simulink model "frequency_measurement_withHELP"  (R2013a)
settings: Solver=ode45  StartTime=0.0  StopTime=0.1  RelTol=1e-3
PreLoadFcn:
  | Freq=[0 150;1 150];
InitFcn:
  | Freq=[0 150;1 150];
  | hit=0.00001;
  | v=.1;
libraries: simulink x1, dspswit3 x1, dspsigops x1
settings Model: Creator=MAT-DEPT  LastModifiedBy=CYBORG
settings DataIOCC: SignalLoggingSaveFormat=ModelDataLogs
settings OptimizationCC: ExpressionDepthLimit=2147483647
settings DebuggingCC: FcnCallInpInsideContextMsg=UseLocalSettings  StrictBusMsg=Warning
settings GRTTargetCC: CombineOutputUpdateFcns=off  GRTInterface=on

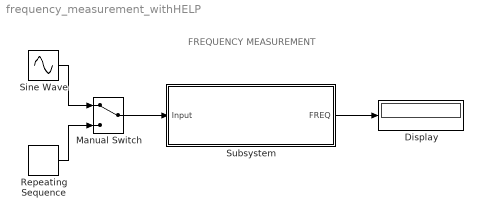
== system frequency_measurement_withHELP ==
  note: FREQUENCY MEASUREMENT
  Display : Display
  Manual Switch : ManualSwitch
  Repeating Sequence : simulink/Sources/Repeating Sequence  rep_seq_t=[0 1/3000]  rep_seq_y=[0 1]
  Sine Wave : Sin  Frequency=2*pi*30  SampleTime=0
  Subsystem : Subsystem  mask(Frequency Measurement){b=External Signal, a=Freq, fo=500, hit=.5, v=0.1}
      mask prompts: b "Type of input:"; a "Workspace Data Identifier:"; fo "Test Frequency fo(Hz)"; hit "Hit value for the Non Zero-Crossing signals:"; v "Time scaling factor:"
      mask help:
      | This block measures the frequency of the input signal, also the workspace signal.
      | User can even check the block using the TEST SIGNAL checkbox.
      mask Help:
      | This block measures the frequency of the input signal, also the workspace signal.
      | User can even check the block using the TEST SIGNAL checkbox.
      | </br>
      | <b></br><h3><u>PARAMETERS</u></h3></b></br>
      | <b><u>Type of input:</u></b></br>
      | <b>1.External Signal:</b>To check the frequency of a external signal, Connect the signal to the 'Input' port of the block.</br>
      | <b></br><u>Workspace Data Identifier</u></b></br>There comes a situation where the model runs too slow. In such sitations or a predefined Workspace data set '2' in <b>Type of input</b> and give the workspace variable name.</br> Model initializes with a workspace variable of 'Freq'. User can specify their own Identifier in <b>Workspace Data Identifier</b></br></br>
      | <b><u>Use TEST SIGNAL</u></b></br>Inorder to test the block check the <b>Use TEST SIGNAL</b> check box.
      | </br><b><u></br>Test Frequency f0(Hz):</u></b></br>Specify the frequency of the test signal in <b>Test Frequency f0(Hz)</b>
      | </br></br><b><u>Hit value for the Non Zero-Crossing signals:</u></b></br>
      | The model uses a zero crossing hit detector with rising edge to count the signal .So if the given input signal is not crossing and rising from zero the counter cannot count the exact cycles. So it is recommended to give the center amplitude value of the given signal to get the proper output.
      | </br></br><i><h2><font color='orange'>Note:</font><font color='brown'> The Frequncy will be found after 1 second, because </br><align='center'><b>Frequency = Number of cycles per second.</b></align></font> </marque></font></h2></i></br>
      mask TypeOptions b: External Signal | Workspace Data | Test Signal
      mask Callback b: b_cb(gcb)
      mask Display:
      | disp('FREQUENCY')
      | port_label('input', 1, 'Input')
      | port_label('output', 1, 'Freq')
  wires:
  Subsystem/1(FREQ) -> Display/1
  Sine Wave/1 -> Manual Switch/1
  Repeating Sequence/1 -> Manual Switch/2
  Manual Switch/1 -> Subsystem/1(Input)

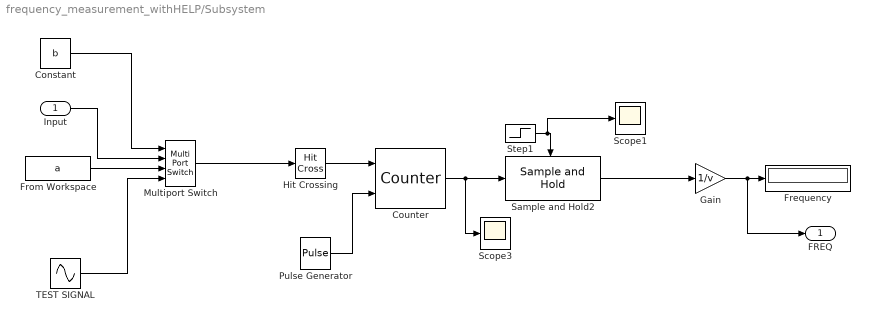
== system frequency_measurement_withHELP/Subsystem ==
  Input : Inport
  Constant : Constant  Value=b
  Counter : dspswit3/Counter  Direction=Up  CountEvent=Rising edge  CounterSize=User defined  MaxCount=10000  InitialCount=0  Output=Count  HitValue=32  ResetInput=on  SamplesPerFrame=1  Ts=1  CntDtype=double  HitDtype=Logical
  "Frequency " : Display
  From Workspace : FromWorkspace  VariableName=a  SampleTime=0
  Gain : Gain  Gain=1/v
  Hit Crossing : HitCross  HitCrossingOffset=hit  HitCrossingDirection=rising
  Multiport Switch : MultiPortSwitch
  Pulse Generator : DiscretePulseGenerator  PulseType=Time based  Period=1  PhaseDelay=v
  Sample and Hold2 : dspsigops/Sample and Hold  trig=Rising edge  initCond=0  latchinput=off
  Scope1 : Scope
      settings: YMin=0  YMax=70  SampleInput=on  SampleTime=5e-6
  Scope3 : Scope
      settings: YMin=0  YMax=70  SampleInput=on  SampleTime=5e-6
  Step1 : Step  Time=v*.99999999  SampleTime=0
  TEST SIGNAL : Sin  Amplitude=10  Frequency=2*pi*fo  SampleTime=0
  FREQ : Outport
  wires:
  Pulse Generator/1 -> Counter/2
  Counter/1 -> Scope3/1, Sample and Hold2/1
  Hit Crossing/1 -> Counter/1
  Step1/1 -> Scope1/1, Sample and Hold2/Trigger
  Sample and Hold2/1 -> Gain/1
  Constant/1 -> Multiport Switch/1
  Input/1 -> Multiport Switch/2
  From Workspace/1 -> Multiport Switch/3
  Gain/1 -> FREQ/1, "Frequency "/1
  TEST SIGNAL/1 -> Multiport Switch/4
  Multiport Switch/1 -> Hit Crossing/1
